simulink model "Custom2ArmRobotFWDKinematicsPID_Controlled"  (R2026a)
settings: Solver=VariableStepAuto  StopTime=4  FixedStep=0.01  RelTol=0.01  AbsTol=0.01  EnableMultiTasking=on
values from neighbouring files (symbols this model uses):
  N = 100    [PlottingOutputPath.m]
undefined symbols (not defined in the file or in its folder): X, Y, Z
libraries: sm_lib x16, nesl_utility x7, slpidlib x2
settings Model: SILPILModeSetting=veronly  ExtModeTrigDuration=2  Creator=acer  LastModifiedBy=acer
settings HardwareCC: ProdBitPerInt=16.0  ProdBitPerPointer=16.0  ProdBitPerSizeT=16.0  ProdBitPerPtrDiffT=16.0  ProdWordSize=8.0  ProdHWDeviceType=Atmel->AVR  UseEmbeddedCoderFeatures=off  UseSimulinkCoderFeatures=off
settings SFSimCC: SimTargetLang=C++
settings RTWCC: SystemTargetFile=ert.tlc  HardwareBoard=Arduino Nano 3.0  TLCOptions=-aInlineSetEventsForThisBaseRateFcn=TLC_FALSE -aSuppressMultiTaskScheduler=TLC_FALSE -aRateBasedStepFcn=1  Toolchain=Arduino AVR  BuildConfiguration=Faster Runs  Description=Embedded Coder
settings ERTTargetCC: ExtModeTransport=3.0  ExtModeAutomaticAllocSize=off  ExtModeStaticAllocSize=250.0  SupportContinuousTime=on  SupportNonInlinedSFcns=on  SupportVariableSizeSignals=on
settings SimscapeCC: SimscapeLogLimitData=off
settings ExplorerConfigSet: InternalSimMechanicsExplorerSettings="<ExplorerConfiguration><canonicalview>default</canonicalview><TilePanel><TileInfo><Tiles Columns=\"1\" Count=\"1\" Height=\"873\" Rows=\"1\" Width=\"1592\"><Row Weight=\"1\"/><Column Weight=\"1\"/><Tile Height=\"1\" Width=\"1\" X=\"0\" Y=\"0\"/></Tiles></TileInfo><SceneInfo><SceneViewer><IsThisViewStd><IsStandardView>off</IsStandardView><StandardViewName>Front</StandardViewName></IsThisViewStd><BGColor><R>1</R><G>1</G><B>1</B><A>1</A></BGColor><Camera><DoPerspective>off</DoPerspective><Position><X>0.66297851591073287</X><Y>-0.55422851665579098</Y><Z>0.69472851593680995</Z></Position><Center><X>0</X><Y>0.10874999925494194</Y><Z>0.03175000002607703</Z></Center><Up><X>-0.40824829046386307</X><Y>0.40824829046386307</Y><Z>0.81649658092772615</Z></Up><XLim>0.12919731782672433</XLim><YLim>0.12919731782672433</YLim><ViewLimDist>0.01</ViewLimDist></Camera></SceneViewer></SceneInfo></TilePanel><MechEditorPanel><GfxPanelCameraMap/><Cameras/><VideoCreator><IncludeTiles>All</IncludeTiles><IncludeTime>on</IncludeTime><IncludeWorldFrame>off</IncludeWorldFrame><PlaybackSpeedRatio>0.5</PlaybackSpeedRatio><FrameRate>30</FrameRate><FrameSize>[1920, 1080]</FrameSize><VideoFormat>UncompressedAVI</VideoFormat></VideoCreator></MechEditorPanel><PlaybackSettings><PlaybackSpeedFactor>1</PlaybackSpeedFactor></PlaybackSettings></ExplorerConfiguration>"

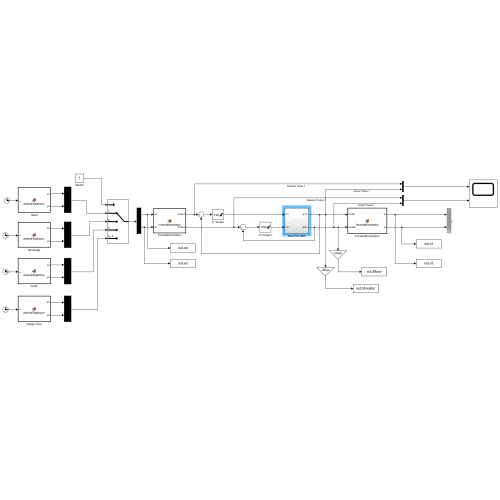
[thumbnail: Simulink's stored preview of the top-level diagram]
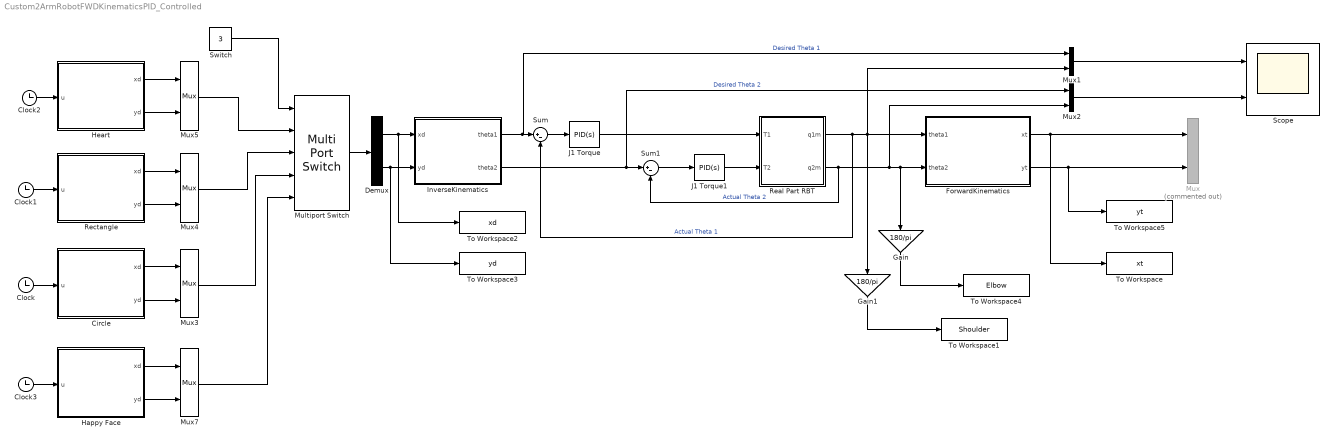
== system Custom2ArmRobotFWDKinematicsPID_Controlled ==
  Circle : MATLAB Function  TreatAsAtomicUnit=on
  Clock{,1..3} (4 alike) : Clock
  Demux : Demux  Outputs=2
  ForwardKinematics : MATLAB Function  TreatAsAtomicUnit=on
  Gain : Gain  Gain=180/pi
  Gain1 : Gain  Gain=180/pi
  Happy Face : MATLAB Function  TreatAsAtomicUnit=on
  Heart : MATLAB Function  TreatAsAtomicUnit=on
  InverseKinematics : MATLAB Function  TreatAsAtomicUnit=on
  J1 Torque : slpidlib/PID Controller  Controller=PID  Form=Parallel  TimeDomain=Continuous-time  UseExternalTs=off  SampleTime=-1  IntegratorMethod=Forward Euler  FilterMethod=Forward Euler  ControllerParametersSource=internal  P=2000  I=120360  UseKiTs=off  D=5  UseExternalDerivativeSource=off  N=3500  UseFilter=on  TunerSelectOption=Transfer Function Based (PID Tuner App)  InitialConditionSource=internal  InitialConditionForIntegrator=0  InitialConditionForFilter=0  DifferentiatorICPrevScaledInput=0  ExternalReset=none  TrackingMode=off  Kt=1  LimitOutput=on  SatLimitsSource=internal  UpperSaturationLimit=inf  LowerSaturationLimit=-inf  LinearizeAsGain=on  AntiWindupMode=clamping  Kb=1  LimitIntegrator=on  UpperIntegratorSaturationLimit=inf  LowerIntegratorSaturationLimit=-inf  POutMin=[]  POutMax=[]  IOutMin=[]  IOutMax=[]  DOutMin=[]  DOutMax=[]  NOutMin=[]  NOutMax=[]  SumOutMin=[]  SumOutMax=[]  SaturationOutMin=[]  SaturationOutMax=[]  PParamMin=[]  PParamMax=[]  IParamMin=[]  IParamMax=[]  DParamMin=[]  DParamMax=[]  NParamMin=[]  NParamMax=[]  KbParamMin=[]  KbParamMax=[]  KtParamMin=[]  KtParamMax=[]  KbOutMin=[]  KbOutMax=[]  KtOutMin=[]  KtOutMax=[]  IntegratorOutMin=[]  IntegratorOutMax=[]  FilterOutMin=[]  FilterOutMax=[]  SumI1OutMin=[]  SumI1OutMax=[]  SumI2OutMin=[]  SumI2OutMax=[]  SumI3OutMin=[]  SumI3OutMax=[]  SumI4OutMin=[]  SumI4OutMax=[]  SumDOutMin=[]  SumDOutMax=[]  DifferentiatorOutMin=[]  DifferentiatorOutMax=[]  FilterDiffOutCoefMin=[]  FilterDiffOutCoefMax=[]  ReciprocalOutMin=[]  ReciprocalOutMax=[]  SumDenOutMin=[]  SumDenOutMax=[]  SumNumOutMin=[]  SumNumOutMax=[]  DivideOutMin=[]  DivideOutMax=[]  UdiffTsProdOutMin=[]  UdiffTsProdOutMax=[]  NTsProdOutMin=[]  NTsProdOutMax=[]  UintegralTsProdOutMin=[]  UintegralTsProdOutMax=[]  UngainTsProdOutMin=[]  UngainTsProdOutMax=[]  ClampingZeroOutDataTypeStr=Inherit: Inherit via back propagation  ClampingZeroOutMin=[]  ClampingZeroOutMax=[]  FilterDenConstantOutDataTypeStr=Inherit: Inherit via back propagation  FilterDenConstantOutMin=[]  FilterDenConstantOutMax=[]  PCopyOutDataTypeStr=Inherit: Inherit via back propagation  PCopyOutMin=[]  PCopyOutMax=[]  NCopyOutDataTypeStr=Inherit: Inherit via back propagation  NCopyOutMin=[]  NCopyOutMax=[]  IntegratorContinuousStateAttributes=''  IntegratorStateMustResolveToSignalObject=off  IntegratorRTWStateStorageClass=Auto  FilterContinuousStateAttributes=''  FilterStateMustResolveToSignalObject=off  FilterRTWStateStorageClass=Auto  ParallelPVariant=InternalParameters  IdealPVariant=Disabled  IVariant=InternalParameters  DVariant=InternalParameters  IntegratorVariant=Continuous  SatVariant=Enabled  AWVariant=ContClampingParallel  PCopyVariant=Disabled  TRVariant=Disabled  FdbkBlocksVariant=Forward  IdealPFdbkVariant=Disabled  SatFdbkVariant=Disabled  DerivativeFilterVariant=ContFilter  NVariant=InternalParameters  NCopyVariant=Disabled  FilterICVariant=InternalICsFilter  IntegratorICVariant=InternalICs  ExternalResetVariant=Disabled  TRSumVariant=Passthrough  SumFdbkVariant=Disabled  SumVariant=Sum_PID  TsampFilterVariant=InternalTs  TsampNgainVariant=Passthrough  TsampIntegralVariant=Disabled_SignalSpec  ExternalSaturationOutDataTypeStr=Inherit: Same as second input  DerivativeSourceVariant=ErrorSignal  PreIntVariant=InternalPreInt
  J1 Torque1 : slpidlib/PID Controller  Controller=PID  Form=Parallel  TimeDomain=Continuous-time  UseExternalTs=off  SampleTime=-1  IntegratorMethod=Forward Euler  FilterMethod=Forward Euler  ControllerParametersSource=internal  P=2000  I=120360  UseKiTs=off  D=5  UseExternalDerivativeSource=off  N=3500  UseFilter=on  TunerSelectOption=Transfer Function Based (PID Tuner App)  InitialConditionSource=internal  InitialConditionForIntegrator=0  InitialConditionForFilter=0  DifferentiatorICPrevScaledInput=0  ExternalReset=none  TrackingMode=off  Kt=1  LimitOutput=on  SatLimitsSource=internal  UpperSaturationLimit=inf  LowerSaturationLimit=-inf  LinearizeAsGain=on  AntiWindupMode=clamping  Kb=1  LimitIntegrator=on  UpperIntegratorSaturationLimit=inf  LowerIntegratorSaturationLimit=-inf  POutMin=[]  POutMax=[]  IOutMin=[]  IOutMax=[]  DOutMin=[]  DOutMax=[]  NOutMin=[]  NOutMax=[]  SumOutMin=[]  SumOutMax=[]  SaturationOutMin=[]  SaturationOutMax=[]  PParamMin=[]  PParamMax=[]  IParamMin=[]  IParamMax=[]  DParamMin=[]  DParamMax=[]  NParamMin=[]  NParamMax=[]  KbParamMin=[]  KbParamMax=[]  KtParamMin=[]  KtParamMax=[]  KbOutMin=[]  KbOutMax=[]  KtOutMin=[]  KtOutMax=[]  IntegratorOutMin=[]  IntegratorOutMax=[]  FilterOutMin=[]  FilterOutMax=[]  SumI1OutMin=[]  SumI1OutMax=[]  SumI2OutMin=[]  SumI2OutMax=[]  SumI3OutMin=[]  SumI3OutMax=[]  SumI4OutMin=[]  SumI4OutMax=[]  SumDOutMin=[]  SumDOutMax=[]  DifferentiatorOutMin=[]  DifferentiatorOutMax=[]  FilterDiffOutCoefMin=[]  FilterDiffOutCoefMax=[]  ReciprocalOutMin=[]  ReciprocalOutMax=[]  SumDenOutMin=[]  SumDenOutMax=[]  SumNumOutMin=[]  SumNumOutMax=[]  DivideOutMin=[]  DivideOutMax=[]  UdiffTsProdOutMin=[]  UdiffTsProdOutMax=[]  NTsProdOutMin=[]  NTsProdOutMax=[]  UintegralTsProdOutMin=[]  UintegralTsProdOutMax=[]  UngainTsProdOutMin=[]  UngainTsProdOutMax=[]  ClampingZeroOutDataTypeStr=Inherit: Inherit via back propagation  ClampingZeroOutMin=[]  ClampingZeroOutMax=[]  FilterDenConstantOutDataTypeStr=Inherit: Inherit via back propagation  FilterDenConstantOutMin=[]  FilterDenConstantOutMax=[]  PCopyOutDataTypeStr=Inherit: Inherit via back propagation  PCopyOutMin=[]  PCopyOutMax=[]  NCopyOutDataTypeStr=Inherit: Inherit via back propagation  NCopyOutMin=[]  NCopyOutMax=[]  IntegratorContinuousStateAttributes=''  IntegratorStateMustResolveToSignalObject=off  IntegratorRTWStateStorageClass=Auto  FilterContinuousStateAttributes=''  FilterStateMustResolveToSignalObject=off  FilterRTWStateStorageClass=Auto  ParallelPVariant=InternalParameters  IdealPVariant=Disabled  IVariant=InternalParameters  DVariant=InternalParameters  IntegratorVariant=Continuous  SatVariant=Enabled  AWVariant=ContClampingParallel  PCopyVariant=Disabled  TRVariant=Disabled  FdbkBlocksVariant=Forward  IdealPFdbkVariant=Disabled  SatFdbkVariant=Disabled  DerivativeFilterVariant=ContFilter  NVariant=InternalParameters  NCopyVariant=Disabled  FilterICVariant=InternalICsFilter  IntegratorICVariant=InternalICs  ExternalResetVariant=Disabled  TRSumVariant=Passthrough  SumFdbkVariant=Disabled  SumVariant=Sum_PID  TsampFilterVariant=InternalTs  TsampNgainVariant=Passthrough  TsampIntegralVariant=Disabled_SignalSpec  ExternalSaturationOutDataTypeStr=Inherit: Same as second input  DerivativeSourceVariant=ErrorSignal  PreIntVariant=InternalPreInt
  Multiport Switch : MultiPortSwitch  Inputs=4  SaturateOnIntegerOverflow=off  InputSameDT=off
  Mux : Mux  Commented=on  Inputs=2
  Mux{1..5,7} (6 alike) : Mux  Inputs=2
  Real Part RBT : Subsystem
  Rectangle : MATLAB Function  TreatAsAtomicUnit=on
  Scope : Scope  NumInputPorts=2
      settings: ActiveDisplayYMinimum=-0.084842773343656835  ActiveDisplayYMaximum=0.76358496009291166  YLabel=Angle (rad)
  Sum : Sum  Inputs=|+-
  Sum1 : Sum  Inputs=|+-
  Switch : Constant  Value=3
  To Workspace : ToWorkspace  VariableName=xt  SaveFormat=Timeseries  SampleTime=-1
  To Workspace1 : ToWorkspace  VariableName=Shoulder  SaveFormat=Timeseries  SampleTime=-1
  To Workspace2 : ToWorkspace  VariableName=xd  SaveFormat=Timeseries  SampleTime=-1
  To Workspace3 : ToWorkspace  VariableName=yd  SaveFormat=Timeseries  SampleTime=-1
  To Workspace4 : ToWorkspace  VariableName=Elbow  SaveFormat=Timeseries  SampleTime=-1
  To Workspace5 : ToWorkspace  VariableName=yt  SaveFormat=Timeseries  SampleTime=-1
  wires:
  Mux1/1 -> Scope/1
  Mux2/1 -> Scope/2
  Clock/1 -> Circle/1(u)
  ForwardKinematics/2(yt) -> To Workspace5/1, Mux/2
  ForwardKinematics/1(xt) -> To Workspace/1, Mux/1
  Clock1/1 -> Rectangle/1(u)
  Multiport Switch/1 -> Demux/1
  Demux/1 -> To Workspace2/1, InverseKinematics/1(xd)
  Demux/2 -> InverseKinematics/2(yd), To Workspace3/1
  Circle/1(xd) -> Mux3/1
  Circle/2(yd) -> Mux3/2
  Mux3/1 -> Multiport Switch/4
  Rectangle/2(yd) -> Mux4/2
  Rectangle/1(xd) -> Mux4/1
  Mux4/1 -> Multiport Switch/3
  Heart/1(xd) -> Mux5/1
  Heart/2(yd) -> Mux5/2
  Mux5/1 -> Multiport Switch/2
  Clock2/1 -> Heart/1(u)
  Switch/1 -> Multiport Switch/1
  Real Part RBT/1(q1m) -> Gain1/1, Mux1/2, ForwardKinematics/1(theta1), Sum/2  "Actual Theta 1"
  Clock3/1 -> Happy Face/1(u)
  Happy Face/1(xd) -> Mux7/1
  Happy Face/2(yd) -> Mux7/2
  J1 Torque1/1 -> Real Part RBT/2(T2)
  Sum1/1 -> J1 Torque1/1
  InverseKinematics/2(theta2) -> Sum1/1, Mux2/1  "Desired Theta 2"
  InverseKinematics/1(theta1) -> Mux1/1, Sum/1  "Desired Theta 1"
  J1 Torque/1 -> Real Part RBT/1(T1)
  Sum/1 -> J1 Torque/1
  Mux7/1 -> Multiport Switch/5
  Real Part RBT/2(q2m) -> Gain/1, ForwardKinematics/2(theta2), Mux2/2, Sum1/2  "Actual Theta 2"
  Gain/1 -> To Workspace4/1
  Gain1/1 -> To Workspace1/1

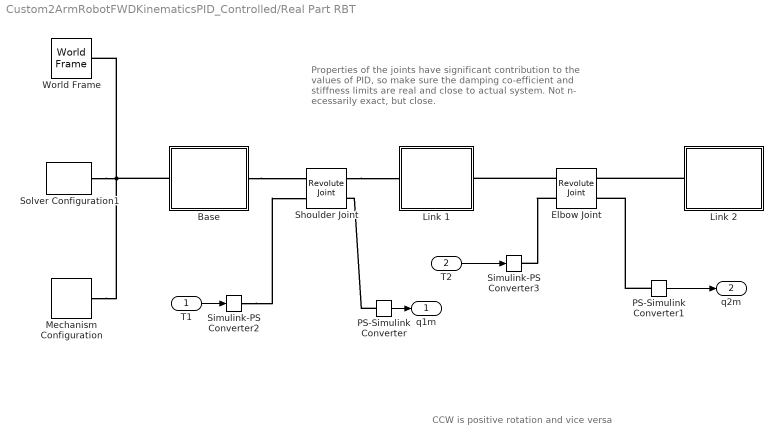
== system Custom2ArmRobotFWDKinematicsPID_Controlled/Real Part RBT ==
  note: Properties of the joints have significant contribution to the
      | values of PID, so make sure the damping co-efficient and
      | stiffness limits are real and close to actual system. Not n-
      | ecessarily exact, but close.
  note: CCW is positive rotation and vice versa
  T1 : Inport
  T2 : Inport  Port=2
  Base : Subsystem
  Elbow Joint : sm_lib/Joints/Revolute Joint  JointMode=Normal  CompositeWrenchDir=FollowerOnBase  CompositeWrenchFrame=BaseFrame  SenseConstraintForce=off  SenseConstraintTorque=off  SenseTotalForce=off  SenseTotalTorque=off  PositionTargetSpecify=on  PositionTargetPriority=High  PositionTargetValue=0  PositionTargetValueUnits=rad  VelocityTargetSpecify=on  VelocityTargetPriority=High  VelocityTargetValue=1  VelocityTargetValueUnits=deg/s  EquilibriumPosition=0  EquilibriumPositionUnits=rad  SpringStiffness=1  SpringStiffnessUnits=N*m/deg  DampingCoefficient=1  DampingCoefficientUnits=N*m/(deg/s)  LowerLimitSpecify=on  LowerLimitBound=0  LowerLimitBoundUnits=rad  LowerLimitStiffness=10  LowerLimitStiffnessUnits=N*m/rad  LowerLimitDamping=10  LowerLimitDampingUnits=N*m*s/rad  LowerLimitTransitionRegionWidth=pi  LowerLimitTransitionRegionWidthUnits=deg  UpperLimitSpecify=on  UpperLimitBound=180  UpperLimitBoundUnits=rad  UpperLimitStiffness=1e2  UpperLimitStiffnessUnits=N*m/rad  UpperLimitDamping=1  UpperLimitDampingUnits=N*m*s/rad  UpperLimitTransitionRegionWidth=pi  UpperLimitTransitionRegionWidthUnits=rad  TorqueActuationMode=InputTorque  MotionActuationMode=ComputedMotion  SensePosition=on  SenseVelocity=off  SenseAcceleration=off  SenseTorqueForce=off  SenseLowerLimitTorqueForce=off  SenseUpperLimitTorqueForce=off
  Link 1 : Subsystem
  Link 2 : Subsystem
  Mechanism Configuration : sm_lib/Utilities/Mechanism Configuration  UniformGravity=Constant  GravityVector=[0 0 -9806.65]  GravityVectorUnits=mm/s^2  LinearizationDelta=0.001  JointModeTransitionNonlinearIterations=2
  PS-Simulink Converter : nesl_utility/PS-Simulink Converter  PhysicalDomain=network_engine_domain  SubClassName=ps_output  LeftPortType=input  RightPortType=output  PseudoPeriodic=off  Frequencies=[]  VectorFormat=inherit  Unit=inherit  AffineConversion=off
  PS-Simulink Converter1 : nesl_utility/PS-Simulink Converter  PhysicalDomain=network_engine_domain  SubClassName=ps_output  LeftPortType=input  RightPortType=output  PseudoPeriodic=off  Frequencies=[]  VectorFormat=inherit  Unit=inherit  AffineConversion=off
  Shoulder Joint : sm_lib/Joints/Revolute Joint  JointMode=Normal  CompositeWrenchDir=FollowerOnBase  CompositeWrenchFrame=BaseFrame  SenseConstraintForce=off  SenseConstraintTorque=off  SenseTotalForce=off  SenseTotalTorque=off  PositionTargetSpecify=on  PositionTargetPriority=High  PositionTargetValue=0  PositionTargetValueUnits=rad  VelocityTargetSpecify=on  VelocityTargetPriority=High  VelocityTargetValue=1  VelocityTargetValueUnits=deg/s  EquilibriumPosition=0  EquilibriumPositionUnits=deg  SpringStiffness=1  SpringStiffnessUnits=N*m/deg  DampingCoefficient=1  DampingCoefficientUnits=N*m/(deg/s)  LowerLimitSpecify=on  LowerLimitBound=0  LowerLimitBoundUnits=rad  LowerLimitStiffness=10  LowerLimitStiffnessUnits=N*m/rad  LowerLimitDamping=10  LowerLimitDampingUnits=N*m*s/rad  LowerLimitTransitionRegionWidth=pi  LowerLimitTransitionRegionWidthUnits=rad  UpperLimitSpecify=on  UpperLimitBound=180  UpperLimitBoundUnits=rad  UpperLimitStiffness=1e2  UpperLimitStiffnessUnits=N*m/rad  UpperLimitDamping=1  UpperLimitDampingUnits=N*m*s/rad  UpperLimitTransitionRegionWidth=0.1  UpperLimitTransitionRegionWidthUnits=rad  TorqueActuationMode=InputTorque  MotionActuationMode=ComputedMotion  SensePosition=on  SenseVelocity=off  SenseAcceleration=off  SenseTorqueForce=off  SenseLowerLimitTorqueForce=off  SenseUpperLimitTorqueForce=off
  Simulink-PS Converter2 : nesl_utility/Simulink-PS Converter  PhysicalDomain=network_engine_domain  SubClassName=ps_input  LeftPortType=input  RightPortType=output  PseudoPeriodic=off  Frequencies=[]  NoiseDistribution=none  NoiseParameters=[]  Unit=N*m  AffineConversion=off  FilteringAndDerivatives=provide  SimscapeFilterOrder=1  InputFilterTimeConstant=0.001  UdotUserProvided=0
  Simulink-PS Converter3 : nesl_utility/Simulink-PS Converter  PhysicalDomain=network_engine_domain  SubClassName=ps_input  LeftPortType=input  RightPortType=output  PseudoPeriodic=off  Frequencies=[]  NoiseDistribution=none  NoiseParameters=[]  Unit=N*m  AffineConversion=off  FilteringAndDerivatives=provide  SimscapeFilterOrder=1  InputFilterTimeConstant=0.001  UdotUserProvided=0
  Solver Configuration1 : nesl_utility/Solver Configuration  PhysicalDomain=network_engine_domain  SubClassName=solver  LeftPortType=input  RightPortType=generic  Tones=[]  Harmonics=[]  SimulateNoise=off  Profile=off  UseLocalSampling=off  EnableSwitchedLinearOptims=on  FrequencyDomain=off  UseCCode=off  RelTol=0.001  AbsTol=0.001  MinStep=1e-09  ToWorkspace=off  RevertToSquareIcSolve=off  NumHomotopyIterations=100  PhasorMode=off  PhasorModeNumHarmonics=1  ConsistencySolver=NEWTON_XTOL_AFTER_FTOL  CanonicalOrdering=CANONICAL  OptimizeIntermediates=OPTIMIZED  IndexReductionMethod=DerivativeReplacement  DoDC=off  ResidualTolerance=1e-09  ConsistencyTolSource=GLOBAL  ConsistencyAbsTol=0.001  ConsistencyRelTol=0.001  ConsistencyTolFactor=0.001  UseLocalSolver=off  LocalSolverChoice=NE_BACKWARD_EULER_ADVANCER  ResolveIndetEquations=on  FunctionEvalNumThread=1  LocalSolverSampleTime=0.001  DoFixedCost=off  MaxNonlinIter=3  MaxModeIter=2  ComputeImpulses=off  ImpulseIterations=2  LinearAlgebra=auto  LinearAlgebraNumThread=0  EquationFormulation=NE_TIME_EF  DelaysMemoryBudget=1024  AutomaticFiltering=on  FilteringTimeConstant=0.001  PartitionStorageMethod=AS_NEEDED  PartitionMemoryBudget=1024  PartitionMethod=ROBUST  MultibodyUseLocalSolver=off  MultibodyLocalSolverChoice=ODE1  MultibodyLocalSolverSampleTime=0.001
  World Frame : sm_lib/Frames and Transforms/World Frame
  q1m : Outport
  q2m : Outport  Port=2
  wires:
  PS-Simulink Converter1/1 -> q2m/1
  PS-Simulink Converter/1 -> q1m/1
  T2/1 -> Simulink-PS Converter3/1
  T1/1 -> Simulink-PS Converter2/1
  connections:
  Shoulder Joint/RConn1 -- Link 1/LConn1
  Elbow Joint/LConn1 -- Link 1/RConn1
  Mechanism Configuration/RConn1 -- Solver Configuration1/RConn1 -- Base/LConn1 -- World Frame/RConn1
  Link 2/LConn1 -- Elbow Joint/RConn1
  PS-Simulink Converter1/LConn1 -- Elbow Joint/RConn2
  Base/RConn1 -- Shoulder Joint/LConn1
  PS-Simulink Converter/LConn1 -- Shoulder Joint/RConn2
  Simulink-PS Converter2/RConn1 -- Shoulder Joint/LConn2
  Elbow Joint/LConn2 -- Simulink-PS Converter3/RConn1

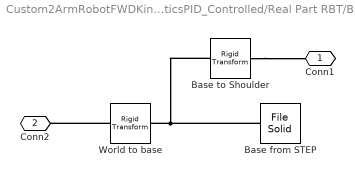
== system Custom2ArmRobotFWDKinematicsPID_Controlled/Real Part RBT/Base ==
  Base from STEP : sm_lib/Body Elements/File Solid  ExtGeomFileName=D:\Desktop\SolidworksSCARA\SimscapeModel\WorkingArmOnly\New_STEP_Assembly\Base.STEP  UnitType=FromFile  ExtGeomFileUnits=m  StepReaderType=HEX  ExportConvexHullGeometry=off  InertiaType=CalculateFromGeometry  BasedOnType=Density  Density=1230  DensityUnits=kg/m^3  Mass=1230  MassUnits=kg  CenterOfMass=[0 0 0]  CenterOfMassUnits=m  MomentsOfInertia=[1 1 1]  MomentsOfInertiaUnits=kg*m^2  ProductsOfInertia=[0 0 0]  ProductsOfInertiaUnits=kg*m^2  GraphicType=FromGeometry  MarkerShape=Sphere  MarkerSize=10  GraphicVisPropType=SimpleVisualProperties  GraphicDiffuseColor=[0.5 0.5 0.5]  GraphicOpacity=1  GraphicSpecularColor=[0.5 0.5 0.5 1.0]  GraphicAmbientColor=[0.15 0.15 0.15 1.0]  GraphicEmissiveColor=[0.0 0.0 0.0 1.0]  GraphicShininess=75  DoExposeReferenceFrame=on  SerializedFrames=<Frames/>
  Base to Shoulder : sm_lib/Frames and Transforms/Rigid Transform  RotationMethod=None  FollAlignAxisA=+X  BaseAlignAxisA=+Y  FollAlignAxisB=+Y  BaseAlignAxisB=+Z  RotationStandardAxis=+Z  RotationAngle=0  RotationAngleUnits=deg  RotationArbitraryAxis=[0 0 1]  RotationSequenceAxes=FollowerAxes  RotationSequence=XYX  RotationSequenceAngles=[0 0 0]  RotationSequenceAnglesUnits=deg  RotationMatrix=[1 0 0;0 1 0;0 0 1]  Quaternion=[1 0 0 0]  TranslationMethod=Cartesian  TranslationCartesianOffset=[0 0 30]  TranslationCartesianOffsetUnits=mm  TranslationStandardAxis=+Z  TranslationStandardOffset=0  TranslationStandardOffsetUnits=m  TranslationROffset=0  TranslationROffsetUnits=m  TranslationThetaOffset=0  TranslationThetaOffsetUnits=deg  TranslationZOffset=0  TranslationZOffsetUnits=m
  World to base : sm_lib/Frames and Transforms/Rigid Transform  RotationMethod=None  FollAlignAxisA=+X  BaseAlignAxisA=+Y  FollAlignAxisB=+Y  BaseAlignAxisB=+Z  RotationStandardAxis=+Z  RotationAngle=0  RotationAngleUnits=deg  RotationArbitraryAxis=[0 0 1]  RotationSequenceAxes=FollowerAxes  RotationSequence=XYX  RotationSequenceAngles=[0 0 0]  RotationSequenceAnglesUnits=deg  RotationMatrix=[1 0 0;0 1 0;0 0 1]  Quaternion=[1 0 0 0]  TranslationMethod=Cartesian  TranslationCartesianOffset=[0 0 0]  TranslationCartesianOffsetUnits=mm  TranslationStandardAxis=+Z  TranslationStandardOffset=0  TranslationStandardOffsetUnits=m  TranslationROffset=0  TranslationROffsetUnits=m  TranslationThetaOffset=0  TranslationThetaOffsetUnits=deg  TranslationZOffset=0  TranslationZOffsetUnits=m
  Conn1 : PMIOPort  Side=Right
  Conn2 : PMIOPort  Port=2  Side=Left
  connections:
  Base to Shoulder/LConn1 -- World to base/RConn1 -- Base from STEP/RConn1
  Base to Shoulder/RConn1 -- Conn1/RConn1
  World to base/LConn1 -- Conn2/RConn1

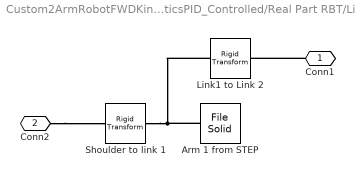
== system Custom2ArmRobotFWDKinematicsPID_Controlled/Real Part RBT/Link 1 ==
  Arm 1 from STEP : sm_lib/Body Elements/File Solid  ExtGeomFileName=D:\Desktop\SolidworksSCARA\SimscapeModel\WorkingArmOnly\New_STEP_Assembly\L1V1.STEP  UnitType=FromFile  ExtGeomFileUnits=m  StepReaderType=HEX  ExportConvexHullGeometry=off  InertiaType=CalculateFromGeometry  BasedOnType=Density  Density=1230  DensityUnits=kg/m^3  Mass=1230  MassUnits=g  CenterOfMass=[0 0 0]  CenterOfMassUnits=m  MomentsOfInertia=[1 1 1]  MomentsOfInertiaUnits=kg*m^2  ProductsOfInertia=[0 0 0]  ProductsOfInertiaUnits=kg*m^2  GraphicType=FromGeometry  MarkerShape=Sphere  MarkerSize=10  GraphicVisPropType=SimpleVisualProperties  GraphicDiffuseColor=[0.5 0.5 0.5]  GraphicOpacity=1  GraphicSpecularColor=[0.5 0.5 0.5 1.0]  GraphicAmbientColor=[0.15 0.15 0.15 1.0]  GraphicEmissiveColor=[0.0 0.0 0.0 1.0]  GraphicShininess=75  DoExposeReferenceFrame=on  SerializedFrames=<Frames/>
  Link1 to Link 2 : sm_lib/Frames and Transforms/Rigid Transform  RotationMethod=None  FollAlignAxisA=+X  BaseAlignAxisA=+Y  FollAlignAxisB=+Y  BaseAlignAxisB=+Z  RotationStandardAxis=+Z  RotationAngle=0  RotationAngleUnits=deg  RotationArbitraryAxis=[0 0 1]  RotationSequenceAxes=FollowerAxes  RotationSequence=XYX  RotationSequenceAngles=[0 0 0]  RotationSequenceAnglesUnits=deg  RotationMatrix=[1 0 0;0 1 0;0 0 1]  Quaternion=[1 0 0 0]  TranslationMethod=Cartesian  TranslationCartesianOffset=[0 130 27.5]  TranslationCartesianOffsetUnits=mm  TranslationStandardAxis=+Z  TranslationStandardOffset=0  TranslationStandardOffsetUnits=m  TranslationROffset=0  TranslationROffsetUnits=m  TranslationThetaOffset=0  TranslationThetaOffsetUnits=deg  TranslationZOffset=0  TranslationZOffsetUnits=m
  Shoulder to link 1 : sm_lib/Frames and Transforms/Rigid Transform  RotationMethod=None  FollAlignAxisA=+X  BaseAlignAxisA=+Y  FollAlignAxisB=+Y  BaseAlignAxisB=+Z  RotationStandardAxis=+Z  RotationAngle=0  RotationAngleUnits=deg  RotationArbitraryAxis=[0 0 1]  RotationSequenceAxes=FollowerAxes  RotationSequence=XYX  RotationSequenceAngles=[0 0 0]  RotationSequenceAnglesUnits=deg  RotationMatrix=[1 0 0;0 1 0;0 0 1]  Quaternion=[1 0 0 0]  TranslationMethod=Cartesian  TranslationCartesianOffset=[0 0 0]  TranslationCartesianOffsetUnits=mm  TranslationStandardAxis=+Z  TranslationStandardOffset=0  TranslationStandardOffsetUnits=m  TranslationROffset=0  TranslationROffsetUnits=m  TranslationThetaOffset=0  TranslationThetaOffsetUnits=deg  TranslationZOffset=0  TranslationZOffsetUnits=m
  Conn1 : PMIOPort  Side=Right
  Conn2 : PMIOPort  Port=2  Side=Left
  connections:
  Conn2/RConn1 -- Shoulder to link 1/LConn1
  Shoulder to link 1/RConn1 -- Link1 to Link 2/LConn1 -- Arm 1 from STEP/RConn1
  Conn1/RConn1 -- Link1 to Link 2/RConn1

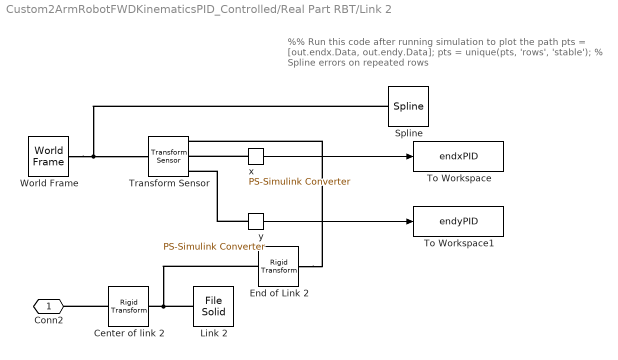
== system Custom2ArmRobotFWDKinematicsPID_Controlled/Real Part RBT/Link 2 ==
  note: %% Run this code after running simulation to plot the path
      | pts = [out.endx.Data, out.endy.Data];
      | pts = unique(pts, 'rows', 'stable');   % Spline errors on repeated rows
  Center of link 2 : sm_lib/Frames and Transforms/Rigid Transform  RotationMethod=None  FollAlignAxisA=+X  BaseAlignAxisA=+Y  FollAlignAxisB=+Y  BaseAlignAxisB=+Z  RotationStandardAxis=+Z  RotationAngle=0  RotationAngleUnits=deg  RotationArbitraryAxis=[0 0 1]  RotationSequenceAxes=FollowerAxes  RotationSequence=XYX  RotationSequenceAngles=[0 0 0]  RotationSequenceAnglesUnits=deg  RotationMatrix=[1 0 0;0 1 0;0 0 1]  Quaternion=[1 0 0 0]  TranslationMethod=Cartesian  TranslationCartesianOffset=[0 0 0]  TranslationCartesianOffsetUnits=mm  TranslationStandardAxis=+Z  TranslationStandardOffset=0  TranslationStandardOffsetUnits=m  TranslationROffset=0  TranslationROffsetUnits=m  TranslationThetaOffset=0  TranslationThetaOffsetUnits=deg  TranslationZOffset=0  TranslationZOffsetUnits=m
  End of Link 2 : sm_lib/Frames and Transforms/Rigid Transform  RotationMethod=None  FollAlignAxisA=+X  BaseAlignAxisA=+Y  FollAlignAxisB=+Y  BaseAlignAxisB=+Z  RotationStandardAxis=+Z  RotationAngle=0  RotationAngleUnits=deg  RotationArbitraryAxis=[0 0 1]  RotationSequenceAxes=FollowerAxes  RotationSequence=XYX  RotationSequenceAngles=[0 0 0]  RotationSequenceAnglesUnits=deg  RotationMatrix=[1 0 0;0 1 0;0 0 1]  Quaternion=[1 0 0 0]  TranslationMethod=Cartesian  TranslationCartesianOffset=[0 130 0]  TranslationCartesianOffsetUnits=mm  TranslationStandardAxis=+Z  TranslationStandardOffset=0  TranslationStandardOffsetUnits=m  TranslationROffset=0  TranslationROffsetUnits=m  TranslationThetaOffset=0  TranslationThetaOffsetUnits=deg  TranslationZOffset=0  TranslationZOffsetUnits=m
  Link 2 : sm_lib/Body Elements/File Solid  ExtGeomFileName=D:\Desktop\SolidworksSCARA\SimscapeModel\WorkingArmOnly\New_STEP_Assembly\L2V1.STEP  UnitType=FromFile  ExtGeomFileUnits=m  StepReaderType=HEX  ExportConvexHullGeometry=off  InertiaType=CalculateFromGeometry  BasedOnType=Density  Density=1230  DensityUnits=kg/m^3  Mass=1230  MassUnits=g  CenterOfMass=[0 0 0]  CenterOfMassUnits=m  MomentsOfInertia=[1 1 1]  MomentsOfInertiaUnits=kg*m^2  ProductsOfInertia=[0 0 0]  ProductsOfInertiaUnits=kg*m^2  GraphicType=FromGeometry  MarkerShape=Sphere  MarkerSize=10  GraphicVisPropType=AdvancedVisualProperties  GraphicDiffuseColor=[1 0.702 0.003922]  GraphicOpacity=1  GraphicSpecularColor=[1 0.702 0.003922]  GraphicAmbientColor=[1 0.702 0.003922]  GraphicEmissiveColor=[0.0 0.0 0.0 1.0]  GraphicShininess=75  DoExposeReferenceFrame=on  SerializedFrames=<Frames/>
  Spline : sm_lib/Curves and Surfaces/Spline  DataPoints=pts_few  DataPointsUnits=m  EndConditionType=Natural  GraphicType=FromGeometry  MarkerShape=Sphere  MarkerSize=10  GraphicVisPropType=SimpleVisualProperties  GraphicDiffuseColor=[0 0 0]  GraphicOpacity=1  GraphicSpecularColor=[0.5 0.5 0.5 1.0]  GraphicAmbientColor=[0.15 0.15 0.15 1.0]  GraphicEmissiveColor=[0.0 0.0 0.0 1.0]  GraphicShininess=75
  To Workspace : ToWorkspace  VariableName=endxPID  SaveFormat=Timeseries  SampleTime=-1
  To Workspace1 : ToWorkspace  VariableName=endyPID  SaveFormat=Timeseries  SampleTime=-1
  Transform Sensor : sm_lib/Frames and Transforms/Transform Sensor  MeasurementFrame=World  RotationSequence=XYX  SenseAngle=off  SenseAxis=off  SenseQ=off  SenseR=off  SenseRotationSequence=off  SenseOmegaX=off  SenseOmegaY=off  SenseOmegaZ=off  SenseOmega=off  SenseQDot=off  SenseRDot=off  SenseRotationSequenceDot=off  SenseAlphaX=off  SenseAlphaY=off  SenseAlphaZ=off  SenseAlpha=off  SenseQDDot=off  SenseRDDot=off  SenseX=on  SenseY=on  SenseZ=off  SenseXYZ=off  SenseRad=off  SenseAzim=off  SenseDist=off  SenseInc=off  SenseXDot=off  SenseYDot=off  SenseZDot=off  SenseXYZDot=off  SenseRadDot=off  SenseAzimDot=off  SenseDistDot=off  SenseIncDot=off  SenseXDDot=off  SenseYDDot=off  SenseZDDot=off  SenseXYZDDot=off  SenseRadDDot=off  SenseAzimDDot=off  SenseDistDDot=off  SenseIncDDot=off
  World Frame : sm_lib/Frames and Transforms/World Frame
  x : nesl_utility/PS-Simulink Converter  PhysicalDomain=network_engine_domain  SubClassName=ps_output  LeftPortType=input  RightPortType=output  PseudoPeriodic=off  Frequencies=[]  VectorFormat=inherit  Unit=inherit  AffineConversion=off
  y : nesl_utility/PS-Simulink Converter  PhysicalDomain=network_engine_domain  SubClassName=ps_output  LeftPortType=input  RightPortType=output  PseudoPeriodic=off  Frequencies=[]  VectorFormat=inherit  Unit=inherit  AffineConversion=off
  Conn2 : PMIOPort  Side=Left
  wires:
  x/1 -> To Workspace/1
  y/1 -> To Workspace1/1
  connections:
  Link 2/RConn1 -- End of Link 2/LConn1 -- Center of link 2/RConn1
  Center of link 2/LConn1 -- Conn2/RConn1
  World Frame/RConn1 -- Spline/LConn1 -- Transform Sensor/LConn1
  x/LConn1 -- Transform Sensor/RConn2
  y/LConn1 -- Transform Sensor/RConn3
  End of Link 2/RConn1 -- Transform Sensor/RConn1

== matlab function Custom2ArmRobotFWDKinematicsPID_Controlled/InverseKinematics ==
  data: theta1 output; theta2 output; xd input; yd input
function [theta1, theta2] = inverseKinematics(xd, yd)
    a1 = 130;
    a2 = 130;

    rSqr = xd^2 + yd^2;
    %r = sqrt(rSqr);

    cosTheta2 = (rSqr - a1^2 - a2^2)/(2*a1*a2);

    %cosTheta2 = min(1, max(-1, cosTheta2)); % clamping angle

    theta2 = -acos(cosTheta2); % elbow angle

    k1 = a1 + a2*cos(theta2);
    k2 = a2 * sin(theta2);

    theta1 = atan2(yd, xd) - atan2(k2, k1);
end

== matlab function Custom2ArmRobotFWDKinematicsPID_Controlled/Circle ==
  data: u input; xd output; yd output
function [xd, yd] = desiredTrajectory(u)
    % Circular path: center (2325,0), diameter 430 (radius 215)
    xc = 233; yc = 0;
    R  = 25;
    T = 4; %Time to complete one circle
    theta = 2*pi*u/T;     % one full revolution as u goes 0 -> 1
    xd = xc + R*cos(theta);
    yd = yc + R*sin(theta);
end

== matlab function Custom2ArmRobotFWDKinematicsPID_Controlled/Heart ==
  data: u input; xd output; yd output
function [xd, yd] = desiredTrajectory(u)
% Heart path: center (233,0), scaled to ~25 units wide
xc = 233; yc = 0;
scale = 1.5;      % adjust to resize the heart (raw curve spans ~32 wide, ~33 tall)
T = 4;           % Time to complete one full loop

theta = 2*pi*u/T;  % one full revolution as u goes 0 -> T

% Classic parametric heart curve
xr = 16*sin(theta)^3;
yr = 13*cos(theta) - 5*cos(2*theta) - 2*cos(3*theta) - cos(4*theta);

xd = xc + scale*xr;
yd = yc + scale*yr;
end

== matlab function Custom2ArmRobotFWDKinematicsPID_Controlled/ForwardKinematics ==
  data: theta1 input; xt output; theta2 input; yt output
function [xt, yt] = forwardKinematics(theta1, theta2)
    a1 = 130; a2 = 130; % arm length
    % xt and yt are position of tip or 2nd arm
    xt = a1 * cos(theta1) + a2 * cos(theta1 + theta2);
    yt = a1 * sin(theta1) + a2 * sin(theta1 + theta2);
end

== matlab function Custom2ArmRobotFWDKinematicsPID_Controlled/Rectangle ==
  data: u input; xd output; yd output
function [xd, yd] = desiredTrajectory(u)
% Rounded-square path: center (xc,yc), side length s, corner fillet radius r
xc = 233; yc = 0;
s  = 50;            % side length
r  = 6;             % corner fillet radius (must be < s/2) — tune this
T  = 4;             % time for one full loop
h  = s/2;

Ls = s - 2*r;            % length of each straight segment
Lc = (pi/2)*r;           % length of each quarter-circle corner
L  = 4*Ls + 4*Lc;        % total perimeter length

v = L / T;               % constant tangential speed (no speed change anywhere)
d = mod(u, T) * v;       % distance traveled along the perimeter, in [0, L)

% Corner arc centers, in traversal order (CCW, starting after bottom-left fillet)
C  = [ xc+h-r, yc-h+r;   % bottom-right corner
       xc+h-r, yc+h-r;   % top-right corner
       xc-h+r, yc+h-r;   % top-left corner
       xc-h+r, yc-h+r ]; % bottom-left corner
a0 = [-pi/2, 0, pi/2, pi];   % starting angle of each corner arc

segLen = [Ls, Lc, Ls, Lc, Ls, Lc, Ls, Lc];
segEnd = cumsum(segLen);

if d < segEnd(1)                 % bottom straight, +x
    xd = (xc - h + r) + d;
    yd = yc - h;
elseif d < segEnd(2)             % bottom-right fillet
    t = d - segEnd(1);  ang = a0(1) + t/r;
    xd = C(1,1) + r*cos(ang);  yd = C(1,2) + r*sin(ang);
elseif d < segEnd(3)             % right straight, +y
    t = d - segEnd(2);
    xd = xc + h;  yd = (yc - h + r) + t;
elseif d < segEnd(4)             % top-right fillet
    t = d - segEnd(3);  ang = a0(2) + t/r;
    xd = C(2,1) + r*cos(ang);  yd = C(2,2) + r*sin(ang);
elseif d < segEnd(5)             % top straight, -x
    t = d - segEnd(4);
    xd = (xc + h - r) - t;  yd = yc + h;
elseif d < segEnd(6)             % top-left fillet
    t = d - segEnd(5);  ang = a0(3) + t/r;
    xd = C(3,1) + r*cos(ang);  yd = C(3,2) + r*sin(ang);
elseif d < segEnd(7)             % left straight, -y
    t = d - segEnd(6);
    xd = xc - h;  yd = (yc + h - r) - t;
else                              % bottom-left fillet
    t = d - segEnd(7);  ang = a0(4) + t/r;
    xd = C(4,1) + r*cos(ang);  yd = C(4,2) + r*sin(ang);
end
end

== matlab function Custom2ArmRobotFWDKinematicsPID_Controlled/Happy Face ==
  data: u input; xd output; yd output
function [xd, yd] = desiredTrajectory(u)
    % Center and bounds: (233,0), fits 50x50 area
    xc = 233; 
    yc = 0;
    T = 10; % Total time to complete the whole face in seconds
    
    % Clamp u to the valid time range [0, T]
    if u > T, u = T; end
    if u < 0, u = 0; end

    % Divide the 4-second timeline into distinct segments
    if u < 1.6
        % 1. Head Outline (0.0s to 1.6s)
        % Map u [0, 1.6] to theta [0, 2*pi]
        theta = (u / 1.6) * 2 * pi;
        xd = xc + 25 * cos(theta);
        yd = yc + 25 * sin(theta);
        
    elseif u < 2.4
        % 2. Left Eye (1.6s to 2.4s)
        % Map u [1.6, 2.4] to theta [0, 2*pi]
        u_local = (u - 1.6) / 0.8;
        theta = u_local * 2 * pi;
        xd = (xc - 8) + 2.5 * cos(theta);
        yd = (yc + 8) + 2.5 * sin(theta);
        
    elseif u < 3.2
        % 3. Right Eye (2.4s to 3.2s)
        % Map u [2.4, 3.2] to theta [0, 2*pi]
        u_local = (u - 2.4) / 0.8;
        theta = u_local * 2 * pi;
        xd = (xc + 8) + 2.5 * cos(theta);
        yd = (yc + 8) + 2.5 * sin(theta);
        
    else
        % 4. Happy Smile (3.2s to 4.0s)
        % Map u [3.2, 4.0] to theta [pi, 2*pi] (semi-circle)
        u_local = (u - 3.2) / 0.8;
        theta = pi + (u_local * pi);
        xd = xc + 12.5 * cos(theta);
        yd = (yc - 2.5) + 12.5 * sin(theta);
    end
end
